simulink model "thd_sim"  (R2019b)
settings: Solver=FixedStepAuto  StartTime=0.0  StopTime=0.06  FixedStep=Ts  RelTol=1e-3
InitFcn:
  | M = readmatrix('MPC_step3_Steady60_300V_THD_tek00028.csv');
  | t = M(16:end,1);
  | Va = M(16:end,2);
  | Vb = M(16:end,4);
  | Vc = M(16:end,3);
  | current = M(16:end,5);
  | Ts = M(3,2);
undefined symbols (not defined in the file or in its folder): plecs
libraries: simulink x4
settings Model: Creator=perei  LastModifiedBy=perei

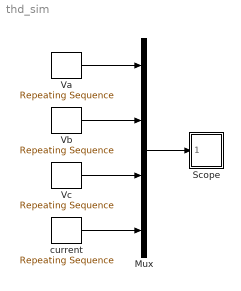
== system thd_sim ==
  Mux : Mux
  Scope : Subsystem  LoadFcn=plecs('sl', 300);  InitFcn=plecs('sl', 314);  StartFcn=plecs('sl', 308);  StopFcn=plecs('sl', 309);  mask{Settings=<binary blob, 1008 chars, not shown>}
      mask init:
      | plecs('sl', 315);
      settings: CopyFcn=plecs('sl', 303);  DeleteFcn=plecs('sl', 305);  UndoDeleteFcn=plecs('sl', 306);  PreSaveFcn=plecs('sl', 311);  NameChangeFcn=plecs('sl', 310);  DestroyFcn=plecs('sl', 307);  OpenFcn=plecs('sl', 302);  ErrorFcn=plerrorfcn
      mask Display: plot([0.1 0.9 0.9 0.1 0.1], [0.9 0.9 0.5 0.5 0.9])
  "Va " : simulink/Sources/Repeating Sequence  rep_seq_t=t  rep_seq_y=Va
  Vb : simulink/Sources/Repeating Sequence  rep_seq_t=t  rep_seq_y=Vb
  Vc : simulink/Sources/Repeating Sequence  rep_seq_t=t  rep_seq_y=Vc
  "current " : simulink/Sources/Repeating Sequence  rep_seq_t=t  rep_seq_y=current
  wires:
  "Va "/1 -> Mux/1
  Vb/1 -> Mux/2
  Vc/1 -> Mux/3
  "current "/1 -> Mux/4
  Mux/1 -> Scope/1(1)

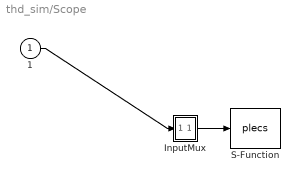
== system thd_sim/Scope ==
  1 : Inport
  " InputMux " : Subsystem
      mask Display: disp('Mux')
  " S-Function " : S-Function  FunctionName=plecs  SFunctionDeploymentMode=off  EnableBusSupport=off
  wires:
  1/1 -> " InputMux "/1(In1)
  " InputMux "/1(Out) -> " S-Function "/1

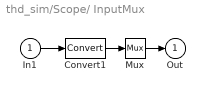
== system thd_sim/Scope/ InputMux  ==
  In1 : Inport
  Convert1 : DataTypeConversion  SaturateOnIntegerOverflow=on  RndMeth=Zero
  Mux : Mux  Inputs=1
  Out : Outport
  wires:
  Convert1/1 -> Mux/1
  In1/1 -> Convert1/1
  Mux/1 -> Out/1
